simulink model "ackerman_modelo_parte2_neuronal"  (R2023b)
settings: Solver=FixedStepDiscrete  StartTime=0.0  StopTime=50  FixedStep=0.1  RelTol=1e-3
undefined symbols (not defined in the file or in its folder): Angular, Linear
libraries: neural x29, robotlib x15, robotcorelib x1
(part 2 of 2)

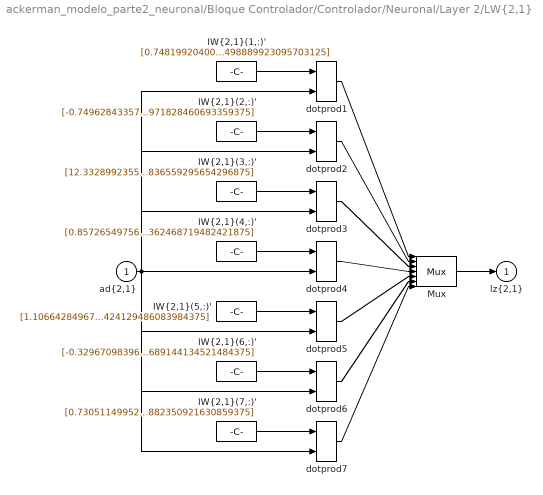
== system ackerman_modelo_parte2_neuronal/Bloque Controlador/Controlador/Neuronal/Layer 2/LW{2,1} ==
  "ad{2,1}" : Inport  PortDimensions=15  SampleTime=0.1
      mask Display: e = 0.06;c1 = [120 230 180]/255;c2 = ([120 230 180]+0)/(256+128);c3 = ([120 230 180]+128)/(256+128);patch([0 1 1 0],[0 0 1 1],c1);patch([0 1 1 1-e 1-e 0+e],[0 0 1 1-e 0+e 0+e],c2);patch([0 0 1 1-e 0+e 0+e],[0 1 1 1-e 1-e 0+e],c3);plot([0 1 1 0 0],[0 0 1 1 0]);
  "IW{2,1}(1,:)'" : Constant  Value=[0.7481992040039153746278088874532841145992279052734375;-1.126597024044754480343044633627869188785552978515625;1.5155775237853175152480389442644082009792327880859375;2.0469156099994307851375197060406208038330078125;7.8138659751533072750362407532520592212677001953125;2.903583859678425138639568103826604783535003662109375;1.6622982814302422749364041010267101228237152099609375;5.9303213640288259256294622900895774364471435546875;-4.31311558360107927256876791943795979022979736328125;-8.8773576403826783831618740805424749851226806640625;-4.04397070113652556955230465973727405071258544921875;-5.08185092549631800551424021250568330287933349609375;-2.80925265953370395521915270364843308925628662109375;-1.864831680495824262067117160768248140811920166015625;2.65513075966677281058991866302676498889923095703125]
      mask Display: e = 0.06;c1 = [120 150 230]/255;c2 = ([120 150 230]+0)/383;c3 = ([120 150 230]+128)/383;patch([0 1 1 0],[0 0 1 1],c1);patch([0 1 1 1-e 1-e 0+e],[0 0 1 1-e 0+e 0+e],c2);patch([0 0 1 1-e 0+e 0+e],[0 1 1 1-e 1-e 0+e],c3);plot([0 1 1 0 0],[0 0 1 1 0]);disp('weights');
  "IW{2,1}(2,:)'" : Constant  Value=[-0.74962843357484931772205527522601187229156494140625;-6.93165936727352960389225700055249035358428955078125;-4.01275508893955379363660540548153221607208251953125;-2.120531649750461600234530123998410999774932861328125;1.829294262234303136693824853864498436450958251953125;6.57831915986466153611900153919123113155364990234375;3.111129228600808982463377105887047946453094482421875;-1.906397126721314894126635408611036837100982666015625;-2.561940433343730116888536940678022801876068115234375;3.701734633273577212975169459241442382335662841796875;2.456765678314351664113246442866511642932891845703125;-0.88958234176935591097645783520420081913471221923828125;-6.4768830231558265353442038758657872676849365234375;4.57889656160470082113533862866461277008056640625;4.0829006341815610170442596427164971828460693359375]
      mask Display: e = 0.06;c1 = [120 150 230]/255;c2 = ([120 150 230]+0)/383;c3 = ([120 150 230]+128)/383;patch([0 1 1 0],[0 0 1 1],c1);patch([0 1 1 1-e 1-e 0+e],[0 0 1 1-e 0+e 0+e],c2);patch([0 0 1 1-e 0+e 0+e],[0 1 1 1-e 1-e 0+e],c3);plot([0 1 1 0 0],[0 0 1 1 0]);disp('weights');
  "IW{2,1}(3,:)'" : Constant  Value=[12.3328992355445858919438251177780330181121826171875;11.0004326759787804945744937867857515811920166015625;-5.34841924221345532686200385796837508678436279296875;-7.0994335148749936337253529927693307399749755859375;2.263077368879132134082965421839617192745208740234375;-7.31242298972578996796300998539663851261138916015625;9.365048931524153630334694753400981426239013671875;3.968973565914051704339726711623370647430419921875;15.059144497544654228704530396498739719390869140625;6.4716573827061711909891528193838894367218017578125;-5.9158271638871067210629917099140584468841552734375;-3.05024650789953444274260618840344250202178955078125;8.2370518811566935113432919024489820003509521484375;-11.6324162769302521525105476030148565769195556640625;2.01322611861408784506011215853504836559295654296875]
      mask Display: e = 0.06;c1 = [120 150 230]/255;c2 = ([120 150 230]+0)/383;c3 = ([120 150 230]+128)/383;patch([0 1 1 0],[0 0 1 1],c1);patch([0 1 1 1-e 1-e 0+e],[0 0 1 1-e 0+e 0+e],c2);patch([0 0 1 1-e 0+e 0+e],[0 1 1 1-e 1-e 0+e],c3);plot([0 1 1 0 0],[0 0 1 1 0]);disp('weights');
  "IW{2,1}(4,:)'" : Constant  Value=[0.85726549756485825870555572691955603659152984619140625;-1.6157874357042329993561224910081364214420318603515625;-2.3378881600398013773656202829442918300628662109375;1.4068312031528831251847577732405625283718109130859375;1.1609880290264327218352491399855352938175201416015625;5.043137081505467023134769988246262073516845703125;1.6282908256337644825606503218295983970165252685546875;0.9851818610864018221917604023474268615245819091796875;-1.5742354980467549996347997876000590622425079345703125;-6.4182878725017058485491361352615058422088623046875;1.236131349069788054606533478363417088985443115234375;-1.5151875690311220612471743152127601206302642822265625;-5.4046776681074533144055749289691448211669921875;-0.301835111587298310364957387719186954200267791748046875;-1.662398546290766443433994936640374362468719482421875]
      mask Display: e = 0.06;c1 = [120 150 230]/255;c2 = ([120 150 230]+0)/383;c3 = ([120 150 230]+128)/383;patch([0 1 1 0],[0 0 1 1],c1);patch([0 1 1 1-e 1-e 0+e],[0 0 1 1-e 0+e 0+e],c2);patch([0 0 1 1-e 0+e 0+e],[0 1 1 1-e 1-e 0+e],c3);plot([0 1 1 0 0],[0 0 1 1 0]);disp('weights');
  "IW{2,1}(5,:)'" : Constant  Value=[1.106642849674602135934264879324473440647125244140625;0.571502015897777937425416894257068634033203125;0.81620295508666396155916800125851295888423919677734375;-3.915085877175725759258284597308374941349029541015625;1.7182548217798458978222697624005377292633056640625;-0.932288532598022801067827458609826862812042236328125;-3.802149167051169786901709812809713184833526611328125;1.1218625349822100023544635405414737761020660400390625;1.2108603063697682689081602802616544067859649658203125;-1.3837647454165533655867648121784441173076629638671875;-2.294782958455342747328131736139766871929168701171875;0.27139709347339202594184826011769473552703857421875;0.35111556880865635310584593753446824848651885986328125;-0.535119520474186316505438298918306827545166015625;0.177795112653033215988074289271025918424129486083984375]
      mask Display: e = 0.06;c1 = [120 150 230]/255;c2 = ([120 150 230]+0)/383;c3 = ([120 150 230]+128)/383;patch([0 1 1 0],[0 0 1 1],c1);patch([0 1 1 1-e 1-e 0+e],[0 0 1 1-e 0+e 0+e],c2);patch([0 0 1 1-e 0+e 0+e],[0 1 1 1-e 1-e 0+e],c3);plot([0 1 1 0 0],[0 0 1 1 0]);disp('weights');
  "IW{2,1}(6,:)'" : Constant  Value=[-0.329670983964105934749255766291753388941287994384765625;0.9447396245833641348355058653396554291248321533203125;-0.260196034449015456413434321802924387156963348388671875;-0.2872857726077722162472127820365130901336669921875;2.91913437532715480671186014660634100437164306640625;0.1852331668108104789638446163735352456569671630859375;0.68985458226234264156317976812715642154216766357421875;-1.7856832233152906130868586842552758753299713134765625;-0.44000187852971850421823774013319052755832672119140625;-2.142873037757759835386650593136437237262725830078125;0.388272349961649665406326903394074179232120513916015625;-0.60718998768551724065645203154417686164379119873046875;0.8371629651469361110827094307751394808292388916015625;0.1650951326068933744384281681050197221338748931884765625;0.64000300449640989963739912127493880689144134521484375]
      mask Display: e = 0.06;c1 = [120 150 230]/255;c2 = ([120 150 230]+0)/383;c3 = ([120 150 230]+128)/383;patch([0 1 1 0],[0 0 1 1],c1);patch([0 1 1 1-e 1-e 0+e],[0 0 1 1-e 0+e 0+e],c2);patch([0 0 1 1-e 0+e 0+e],[0 1 1 1-e 1-e 0+e],c3);plot([0 1 1 0 0],[0 0 1 1 0]);disp('weights');
  "IW{2,1}(7,:)'" : Constant  Value=[0.73051149952431082557069430549745447933673858642578125;3.05826356477004512868234087363816797733306884765625;-1.673669437076252819451838149689137935638427734375;-2.400459004009674490731640617013908922672271728515625;-9.80319466489697077804521541111171245574951171875;4.62435712954842959021561910049058496952056884765625;-4.84177000897603448947847937233746051788330078125;-8.425474797648991653886696440167725086212158203125;-3.37578421790337568353379538166336715221405029296875;-3.11041385548329518684340655454434454441070556640625;2.677786696924715936773964131134562194347381591796875;3.9061912060113375133596491650678217411041259765625;1.013606829036505008190260923583991825580596923828125;4.45431275129676151891544577665627002716064453125;-10.9998218846045059393645715317688882350921630859375]
      mask Display: e = 0.06;c1 = [120 150 230]/255;c2 = ([120 150 230]+0)/383;c3 = ([120 150 230]+128)/383;patch([0 1 1 0],[0 0 1 1],c1);patch([0 1 1 1-e 1-e 0+e],[0 0 1 1-e 0+e 0+e],c2);patch([0 0 1 1-e 0+e 0+e],[0 1 1 1-e 1-e 0+e],c3);plot([0 1 1 0 0],[0 0 1 1 0]);disp('weights');
  Mux : Mux  Inputs=7
      mask Display: e = 0.06;c1 = [120 150 230]/255;c2 = ([120 150 230]+0)/383;c3 = ([120 150 230]+128)/383;patch([0 1 1 0],[0 0 1 1],c1);patch([0 1 1 1-e 1-e 0+e],[0 0 1 1-e 0+e 0+e],c2);patch([0 0 1 1-e 0+e 0+e],[0 1 1 1-e 1-e 0+e],c3);plot([0 1 1 0 0],[0 0 1 1 0]);disp('Mux');
  dotprod{1..7} (7 alike) : neural/Weight Functions/dotprod
  "lz{2,1}" : Outport
      mask Display: e = 0.06;c1 = [120 230 180]/255;c2 = ([120 230 180]+0)/(256+128);c3 = ([120 230 180]+128)/(256+128);patch([0 1 1 0],[0 0 1 1],c1);patch([0 1 1 1-e 1-e 0+e],[0 0 1 1-e 0+e 0+e],c2);patch([0 0 1 1-e 0+e 0+e],[0 1 1 1-e 1-e 0+e],c3);plot([0 1 1 0 0],[0 0 1 1 0]);
  wires:
  Mux/1 -> "lz{2,1}"/1
  dotprod7/1 -> Mux/7
  "IW{2,1}(7,:)'"/1 -> dotprod7/1
  dotprod6/1 -> Mux/6
  "IW{2,1}(6,:)'"/1 -> dotprod6/1
  dotprod5/1 -> Mux/5
  "IW{2,1}(5,:)'"/1 -> dotprod5/1
  dotprod4/1 -> Mux/4
  "IW{2,1}(4,:)'"/1 -> dotprod4/1
  dotprod3/1 -> Mux/3
  "IW{2,1}(3,:)'"/1 -> dotprod3/1
  dotprod2/1 -> Mux/2
  "IW{2,1}(2,:)'"/1 -> dotprod2/1
  dotprod1/1 -> Mux/1
  "ad{2,1}"/1 -> dotprod7/2, dotprod6/2, dotprod5/2, dotprod4/2, dotprod3/2, dotprod2/2, dotprod1/2
  "IW{2,1}(1,:)'"/1 -> dotprod1/1

== system ackerman_modelo_parte2_neuronal/Bloque Controlador/Controlador/Neuronal/Layer 3/Delays 1 ==
  "p{3}" : Inport  PortDimensions=7  SampleTime=0.1
      mask Display: e = 0.06;c1 = [120 230 180]/255;c2 = ([120 230 180]+0)/(256+128);c3 = ([120 230 180]+128)/(256+128);patch([0 1 1 0],[0 0 1 1],c1);patch([0 1 1 1-e 1-e 0+e],[0 0 1 1-e 0+e 0+e],c2);patch([0 0 1 1-e 0+e 0+e],[0 1 1 1-e 1-e 0+e],c3);plot([0 1 1 0 0],[0 0 1 1 0]);
  mux : Mux  Inputs=1
      mask Display: e = 0.06;c1 = [120 150 230]/255;c2 = ([120 150 230]+0)/383;c3 = ([120 150 230]+128)/383;patch([0 1 1 0],[0 0 1 1],c1);patch([0 1 1 1-e 1-e 0+e],[0 0 1 1-e 0+e 0+e],c2);patch([0 0 1 1-e 0+e 0+e],[0 1 1 1-e 1-e 0+e],c3);plot([0 1 1 0 0],[0 0 1 1 0]);disp('Mux')
  "pd{3,2}" : Outport
      mask Display: e = 0.06;c1 = [120 230 180]/255;c2 = ([120 230 180]+0)/(256+128);c3 = ([120 230 180]+128)/(256+128);patch([0 1 1 0],[0 0 1 1],c1);patch([0 1 1 1-e 1-e 0+e],[0 0 1 1-e 0+e 0+e],c2);patch([0 0 1 1-e 0+e 0+e],[0 1 1 1-e 1-e 0+e],c3);plot([0 1 1 0 0],[0 0 1 1 0]);
  wires:
  mux/1 -> "pd{3,2}"/1
  "p{3}"/1 -> mux/1

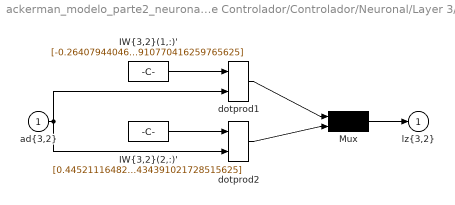
== system ackerman_modelo_parte2_neuronal/Bloque Controlador/Controlador/Neuronal/Layer 3/LW{3,2} ==
  "ad{3,2}" : Inport  PortDimensions=7  SampleTime=0.1
      mask Display: e = 0.06;c1 = [120 230 180]/255;c2 = ([120 230 180]+0)/(256+128);c3 = ([120 230 180]+128)/(256+128);patch([0 1 1 0],[0 0 1 1],c1);patch([0 1 1 1-e 1-e 0+e],[0 0 1 1-e 0+e 0+e],c2);patch([0 0 1 1-e 0+e 0+e],[0 1 1 1-e 1-e 0+e],c3);plot([0 1 1 0 0],[0 0 1 1 0]);
  "IW{3,2}(1,:)'" : Constant  Value=[-0.264079440465544046379164910831605084240436553955078125;0.51230046191857103732303357901400886476039886474609375;-0.6652775182707999501730000702082179486751556396484375;-0.53484339021644611289474369186791591346263885498046875;-0.149228947666670774818697964292368851602077484130859375;-0.008433135735000978072672950247579137794673442840576171875;-0.85256293215924350281653687488869763910770416259765625]
      mask Display: e = 0.06;c1 = [120 150 230]/255;c2 = ([120 150 230]+0)/383;c3 = ([120 150 230]+128)/383;patch([0 1 1 0],[0 0 1 1],c1);patch([0 1 1 1-e 1-e 0+e],[0 0 1 1-e 0+e 0+e],c2);patch([0 0 1 1-e 0+e 0+e],[0 1 1 1-e 1-e 0+e],c3);plot([0 1 1 0 0],[0 0 1 1 0]);disp('weights');
  "IW{3,2}(2,:)'" : Constant  Value=[0.445211164821717797490663315329584293067455291748046875;0.2497172286753712444618003019058960489928722381591796875;0.24675394014089579997062173788435757160186767578125;-0.017453169559885635397922243328139302320778369903564453125;-0.534125695750038431697248597629368305206298828125;0.041939997232147328831697308260118006728589534759521484375;0.475153394142820373335922568003297783434391021728515625]
      mask Display: e = 0.06;c1 = [120 150 230]/255;c2 = ([120 150 230]+0)/383;c3 = ([120 150 230]+128)/383;patch([0 1 1 0],[0 0 1 1],c1);patch([0 1 1 1-e 1-e 0+e],[0 0 1 1-e 0+e 0+e],c2);patch([0 0 1 1-e 0+e 0+e],[0 1 1 1-e 1-e 0+e],c3);plot([0 1 1 0 0],[0 0 1 1 0]);disp('weights');
  Mux : Mux  Inputs=2
      mask Display: e = 0.06;c1 = [120 150 230]/255;c2 = ([120 150 230]+0)/383;c3 = ([120 150 230]+128)/383;patch([0 1 1 0],[0 0 1 1],c1);patch([0 1 1 1-e 1-e 0+e],[0 0 1 1-e 0+e 0+e],c2);patch([0 0 1 1-e 0+e 0+e],[0 1 1 1-e 1-e 0+e],c3);plot([0 1 1 0 0],[0 0 1 1 0]);disp('Mux');
  dotprod1 : neural/Weight Functions/dotprod
  dotprod2 : neural/Weight Functions/dotprod
  "lz{3,2}" : Outport
      mask Display: e = 0.06;c1 = [120 230 180]/255;c2 = ([120 230 180]+0)/(256+128);c3 = ([120 230 180]+128)/(256+128);patch([0 1 1 0],[0 0 1 1],c1);patch([0 1 1 1-e 1-e 0+e],[0 0 1 1-e 0+e 0+e],c2);patch([0 0 1 1-e 0+e 0+e],[0 1 1 1-e 1-e 0+e],c3);plot([0 1 1 0 0],[0 0 1 1 0]);
  wires:
  Mux/1 -> "lz{3,2}"/1
  dotprod2/1 -> Mux/2
  "IW{3,2}(2,:)'"/1 -> dotprod2/1
  dotprod1/1 -> Mux/1
  "ad{3,2}"/1 -> dotprod2/2, dotprod1/2
  "IW{3,2}(1,:)'"/1 -> dotprod1/1

== matlab function ackerman_modelo_parte2_neuronal/ROS Robot/Conversion_diff_ackerman ==
  data: steering_wheel_angle input; V output; linear_vel_ackerman_kmh input; W output
function [V,W] = fcn(steering_wheel_angle, linear_vel_ackerman_kmh)

    %Aproximacion de angulo volante y velocidad linal a vel_linar y angular.
    % *************************************
    
    min_turning_radius_vehicle = 2;  % radio de giro del vehiculo. Radio minimo en el que gira 180 grados. 
    max_turning_radius_vehicle = 34; % radio de giro del vehiculo. Radio máximo con el volante girado 1º
    max_steering_wheel_angle = 90;  % angulo máximo de volante permitido (grados).
    max_vehicle_linear_speed = 30;  % velocidad máxima de vehiculo (km/h).
    
    
    % Filtrado des los valores máximos
    
    if steering_wheel_angle > max_steering_wheel_angle
        steering_wheel_angle = max_steering_wheel_angle;  
    end
    
    if steering_wheel_angle < (-1*max_steering_wheel_angle)
        steering_wheel_angle = max_steering_wheel_angle;  
    end
    
    if linear_vel_ackerman_kmh > max_vehicle_linear_speed
        linear_vel_ackerman_kmh = max_vehicle_linear_speed;
    end
    
    
    %Conversion a m/s
    linear_vel_ackerman_ms = linear_vel_ackerman_kmh/3.6; %(m/s)
    
    %Conversion a linear and angular velocity for the simulator.
    % v=rω --> ω = v/r
    
    % max_steering_wheel_angle -- > min_turning_radius_vehicle
    % steering_wheel_angle = 0 --> angular_vel_vehicle = 0;
    
    turning_radius = (max_turning_radius_vehicle-((max_turning_radius_vehicle-min_turning_radius_vehicle)/max_steering_wheel_angle)*abs(steering_wheel_angle));
    
    if steering_wheel_angle > 0
            turning_radius = turning_radius;
    elseif steering_wheel_angle < 0
            turning_radius = -1*turning_radius;
    end
    
    if abs(steering_wheel_angle) < 0.01
        angular_vel_vehicle = 0;
    else
        angular_vel_vehicle = linear_vel_ackerman_ms / turning_radius;
    end
    
    %Sin velocidad linear, tampoco debe girar
    
    if linear_vel_ackerman_ms == 0
        angular_vel_vehicle = 0;
    end
    
    
    %Rellenamos los campos del mensaje V y W
    V= linear_vel_ackerman_ms;

    W=angular_vel_vehicle;
    
    
    %********************************************************

== matlab function ackerman_modelo_parte2_neuronal/ROS Robot/MATLAB Function ==
  data: u input; y output
function y = fcn(u)
u(isinf(u))=5.0;
y = u;

== matlab function ackerman_modelo_parte2_neuronal/Condicion de Parada ==
  data: flag_parada output; raw_speed input; filter_speed output; sonar_2 input; sonar_3 input; sonar_8 input; sonar_9 input
function [flag_parada, filter_speed] = condicion_parada(raw_speed, sonar_2, sonar_3, sonar_8, sonar_9)

% Condicion de parada:
% - debeis decidir cuando se finaliza la maniobra de aparcamiento en base
%  a la información disponible:
%      - velocidad_lineal
%      - ángulo de volante      
%      - sensores
% Una vez que decidais cual es el criterio de parada debeis:
%   - Parar el vehículo con v_lineal = 0.
%   - Activar el flag_parada a 1 para indicar que ha finalizado la maniobra.

if sonar_2 >= 4 && sonar_3 >= 4 && sonar_8 < 1.3 && sonar_9 < 1.3 % Ejemplo de condición de parada

    %Es necesario parar el vehículo con v_lineal = 0 y activar el
    %flag_parada a 1 para indicar que ha finalizado la maniobra.
    filter_speed = 0.0;
    flag_parada=1;

else
    filter_speed = raw_speed;
    flag_parada=0;
end

== matlab function ackerman_modelo_parte2_neuronal/Evaluacion_maniobra/Evaluacion_fin_maniobra ==
  data: clock input; flag_parada input; x input; y input; theta input; stop_flag output
function stop_flag = evaluacion_maniobra(clock, flag_parada, x, y, theta)

if flag_parada == 1

    parking_time = clock
    parking_position_x = x
    parking_position_y = y
    parking_position_theta = theta
    stop_flag = 1;
else
    stop_flag = 0;

end
